simulink model "calcul_vitesse_yawrate"  (R2024b)
settings: Solver=FixedStepAuto  StartTime=0.0  StopTime=10.0  FixedStep=Ts  RelTol=1e-3
values from neighbouring files (symbols this model uses):
  Izz = 120    [main_data_vehicle.m]
  m = 275    [main_data_vehicle.m]
  Ts = 0.001    [main_data_vehicle.m]
  v0 = 10    [main_data_vehicle.m]
settings Model: Creator=marti  LastModifiedBy=marti

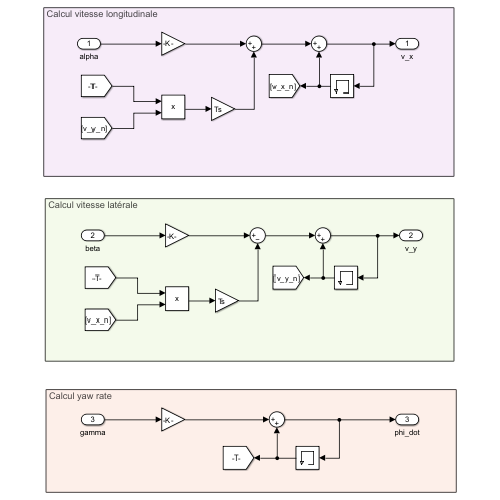
[thumbnail: Simulink's stored preview of the top-level diagram]
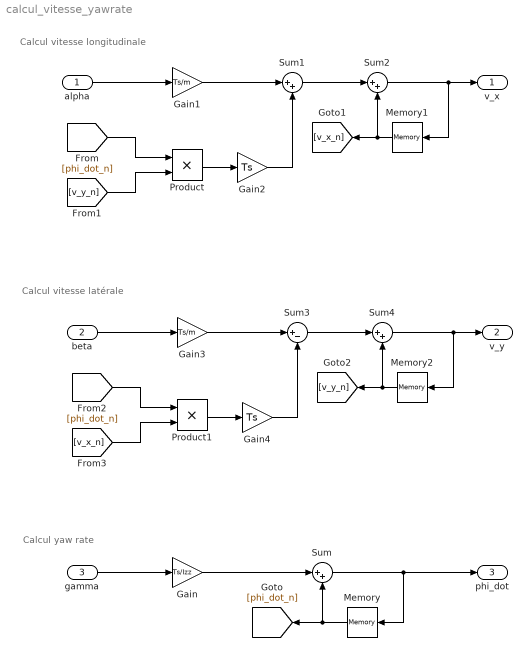
== system calcul_vitesse_yawrate ==
  note: Calcul vitesse latérale
  note: Calcul vitesse longitudinale
  note: Calcul yaw rate
  alpha : Inport
  beta : Inport  Port=2
  gamma : Inport  Port=3
  Gain : Gain  Gain=Ts/Izz
  Gain1 : Gain  Gain=Ts/m
  Gain2 : Gain  Gain=Ts
  Gain3 : Gain  Gain=Ts/m
  Gain4 : Gain  Gain=Ts
  Memory : Memory
  Memory1 : Memory  InitialCondition=v0
  Memory2 : Memory
  Product : Product
  Product1 : Product
  Sum{,1..2,4} (4 alike) : Sum  Inputs=|++
  Sum3 : Sum  Inputs=|+-
  v_x : Outport
  v_y : Outport  Port=2
  phi_dot : Outport  Port=3
  wires:
  alpha/1 -> Gain1/1
  [phi_dot_n] -> Product/1
  [v_y_n] -> Product/2
  Product/1 -> Gain2/1
  Gain1/1 -> Sum1/1
  Gain2/1 -> Sum1/2
  Sum1/1 -> Sum2/1
  Sum2/1 -> Memory1/1, v_x/1
  Memory1/1 -> [v_x_n], Sum2/2
  Gain4/1 -> Sum3/2
  Gain3/1 -> Sum3/1
  [v_x_n] -> Product1/2
  beta/1 -> Gain3/1
  Sum3/1 -> Sum4/1
  [phi_dot_n] -> Product1/1
  Sum4/1 -> Memory2/1, v_y/1
  Memory2/1 -> [v_y_n], Sum4/2
  Product1/1 -> Gain4/1
  Sum/1 -> phi_dot/1, Memory/1
  Gain/1 -> Sum/1
  gamma/1 -> Gain/1
  Memory/1 -> [phi_dot_n], Sum/2
